simulink model "ager"  (R2018b)
settings: Solver=VariableStepAuto  StartTime=0.0  StopTime=100000*3600  RelTol=1e-3
values from neighbouring files (symbols this model uses):
  alpha_batt = 6.87e-07    [ini.m]
  Batt_C = 4    [ini.m]
  beta_batt = 0.02715    [ini.m]
settings Model: Creator=Pedro  LastModifiedBy=Pedro

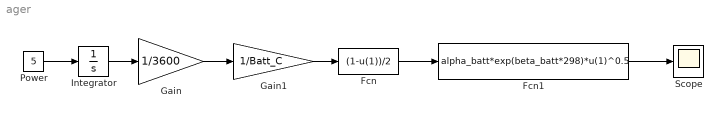
== system ager ==
  Fcn : Fcn  Expr=(1-u(1))/2
  Fcn1 : Fcn  Expr=alpha_batt*exp(beta_batt*298)*u(1)^0.5
  Gain : Gain  Gain=1/3600
  Gain1 : Gain  Gain=1/Batt_C
  Integrator : Integrator
  Power : Constant  Value=5
  Scope : Scope
  wires:
  Power/1 -> Integrator/1
  Gain/1 -> Gain1/1
  Integrator/1 -> Gain/1
  Gain1/1 -> Fcn/1
  Fcn/1 -> Fcn1/1
  Fcn1/1 -> Scope/1
